simulink model "Rate_Adapating_Testing"  (R2023b)
settings: Solver=FixedStepAuto  StartTime=0.0  StopTime=30  FixedStep=1e-3  RelTol=1e-3  EnableMultiTasking=on
libraries: dspstat3 x3, frdmk64flib x1
settings Model: SimulationMode=external  ExtModeTrigDuration=5  Creator=Jeff  LastModifiedBy=conno
settings SolverCC: AlgebraicLoopSolver=TrustRegion
settings OptimizationCC: EnhancedBackFolding=on  PassReuseOutputArgsAs=Individual arguments  ZeroExternalMemoryAtStartup=off  ZeroInternalMemoryAtStartup=off  MaxStackSize=64  OptimizeBlockOrder=speed  DifferentSizesBufferReuse=on  OptimizationCustomize=off  EfficientTunableParamExpr=on
settings DebuggingCC: ParameterTunabilityLossMsg=error  UnconnectedInputMsg=warning  UnconnectedOutputMsg=warning  UnconnectedLineMsg=warning
settings HardwareCC: ProdBitPerPointer=32  ProdBitPerSizeT=32  ProdBitPerPtrDiffT=32  ProdLargestAtomicInteger=Long  ProdLargestAtomicFloat=Double  ProdWordSize=32  ProdHWDeviceType=ARM Compatible->ARM Cortex
settings ModelReferenceCC: EnableRefExpFcnMdlSchedulingChecks=on
settings SFSimCC: MATLABDynamicMemAlloc=off
settings RTWCC: Description=Embedded Coder  SystemTargetFile=ert.tlc  HardwareBoard=NXP FRDM-K64F  TLCOptions="-aInlineSetEventsForThisBaseRateFcn=TLC_FALSE -aSuppressMultiTaskScheduler=TLC_FALSE  -aRateBasedStepFcn=0"  TemplateMakefile=ert_default_tmf  Toolchain=GNU Tools for ARM Embedded Processors
settings CodeAppCC: ForceParamTrailComments=on  IgnoreCustomStorageClasses=off  OperatorAnnotations=on  SimulinkDataObjDesc=on  SFDataObjDesc=on  InsertBlockDesc=on
settings ERTTargetCC: ExtMode=on  ExtModeTransport=4  ExtModeMexFile=sendToCommService  ExtModeMexArgs='tutorial4_3DM4' 0

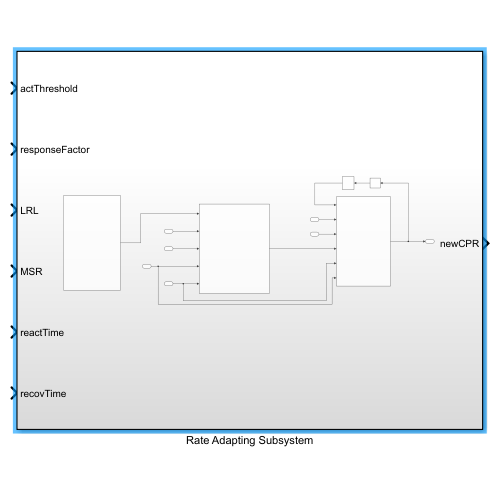
[thumbnail: Simulink's stored preview of the top-level diagram]
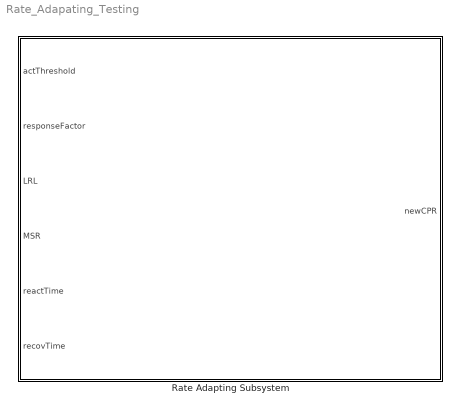
== system Rate_Adapating_Testing ==
  Rate Adapting Subsystem : Subsystem

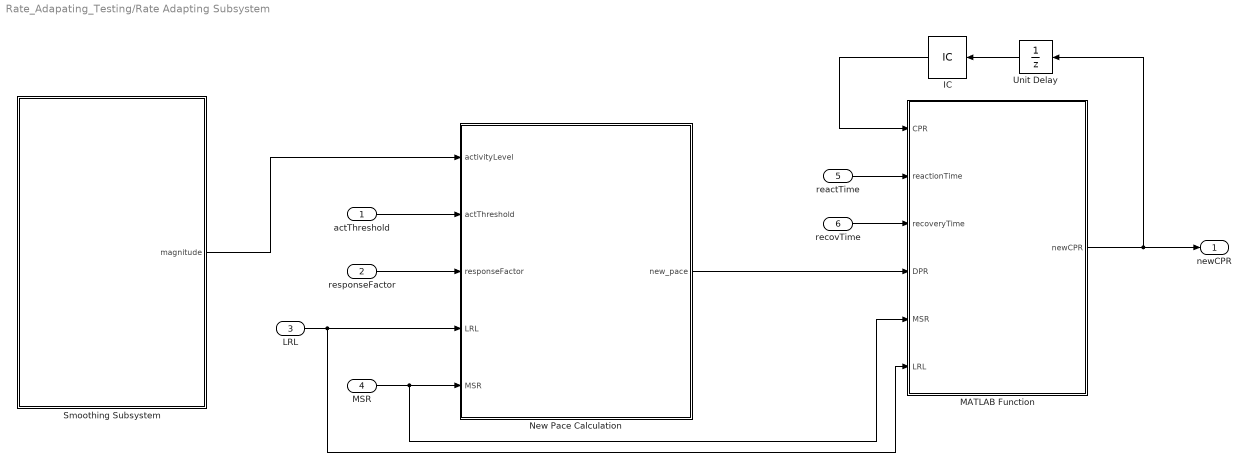
== system Rate_Adapating_Testing/Rate Adapting Subsystem ==
  actThreshold : Inport
  responseFactor : Inport  Port=2
  LRL : Inport  Port=3
  MSR : Inport  Port=4
  reactTime : Inport  Port=5
  recovTime : Inport  Port=6
  IC : InitialCondition  Value=60
  MATLAB Function : MATLAB Function  TreatAsAtomicUnit=on
  New Pace Calculation : MATLAB Function  TreatAsAtomicUnit=on
  Smoothing Subsystem : Subsystem
  Unit Delay : UnitDelay  SampleTime=-1  HasFrameUpgradeWarning=on
  newCPR : Outport
  wires:
  New Pace Calculation/1(new_pace) -> MATLAB Function/4(DPR)
  LRL/1 -> New Pace Calculation/4(LRL), MATLAB Function/6(LRL)
  responseFactor/1 -> New Pace Calculation/3(responseFactor)
  MSR/1 -> New Pace Calculation/5(MSR), MATLAB Function/5(MSR)
  Smoothing Subsystem/1(magnitude) -> New Pace Calculation/1(activityLevel)
  actThreshold/1 -> New Pace Calculation/2(actThreshold)
  MATLAB Function/1(newCPR) -> Unit Delay/1, newCPR/1
  reactTime/1 -> MATLAB Function/2(reactionTime)
  recovTime/1 -> MATLAB Function/3(recoveryTime)
  Unit Delay/1 -> IC/1
  IC/1 -> MATLAB Function/1(CPR)

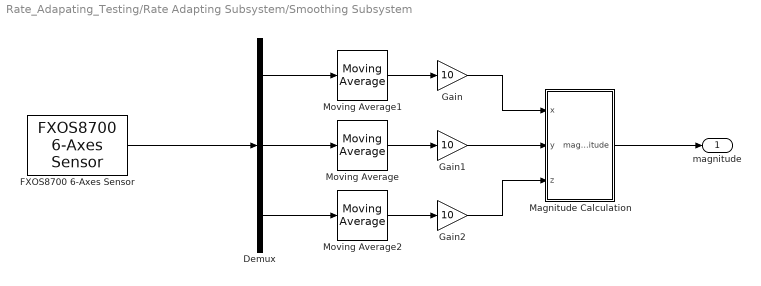
== system Rate_Adapating_Testing/Rate Adapting Subsystem/Smoothing Subsystem ==
  " Magnitude Calculation" : MATLAB Function  TreatAsAtomicUnit=on
  Demux : Demux  Outputs=3
  FXOS8700 6-Axes Sensor : frdmk64flib/FXOS8700 6-Axes Sensor  Activesensor=Accelerometer only  ODR=800Hz  HybridODR=400Hz  Accelfullrange=-4g to +4g  SampleTime=-1
  Gain : Gain  Gain=10
  Gain1 : Gain  Gain=10
  Gain2 : Gain  Gain=10
  Moving Average : dspstat3/Moving Average  Method=Sliding window  ForgettingFactorPort=off  SpecifyWindowLength=on  WindowLength=4  OverlapLength=3  AllowArbitraryInputLength=off  ForgettingFactor=0.9  SimulateUsing=Code generation
  Moving Average1 : dspstat3/Moving Average  Method=Sliding window  ForgettingFactorPort=off  SpecifyWindowLength=on  WindowLength=4  OverlapLength=3  AllowArbitraryInputLength=off  ForgettingFactor=0.9  SimulateUsing=Code generation
  Moving Average2 : dspstat3/Moving Average  Method=Sliding window  ForgettingFactorPort=off  SpecifyWindowLength=on  WindowLength=4  OverlapLength=3  AllowArbitraryInputLength=off  ForgettingFactor=0.9  SimulateUsing=Code generation
  magnitude : Outport
  wires:
  Demux/2 -> Moving Average/1
  Moving Average/1 -> Gain1/1
  Gain/1 -> " Magnitude Calculation"/1(x)
  Demux/1 -> Moving Average1/1
  Gain2/1 -> " Magnitude Calculation"/3(z)
  Moving Average1/1 -> Gain/1
  Demux/3 -> Moving Average2/1
  Gain1/1 -> " Magnitude Calculation"/2(y)
  FXOS8700 6-Axes Sensor/1 -> Demux/1
  Moving Average2/1 -> Gain2/1
  " Magnitude Calculation"/1(magnitude) -> magnitude/1

== matlab function Rate_Adapating_Testing/Rate Adapting Subsystem/New Pace Calculation ==
  data: activityLevel input; actThreshold input; responseFactor input; LRL input; MSR input; new_pace output
function new_pace  = newPace(activityLevel, actThreshold, responseFactor, LRL, MSR)

%Initilization Block
%---------------------------------------------------------------------------------------------------------------------------------------------------
%Acceleration Range of Change
gain = 10; % This is the gain block in the accelorometer
ATMax = sqrt((4*gain)^2+(4*gain)^2+(4*gain)^2)-1; 

%To ensure the pacemaker is static, we remove 1g (gravity)
%Different activity levels listed as strings
actThreshLvl = {'V-Low', 'Low', 'Med-Low', 'Med', 'Med-High', 'High', 'V-High'}; 


%To ensure the percentage is higher than the default 1g, we add 1
%Different activity percentages listed in the same order above
actThreshRange = [0.05*ATMax+1, 0.15*ATMax+1, 0.30*ATMax+1, 0.45*ATMax+1, 0.60*ATMax+1, 0.75*ATMax+1, 0.90*ATMax+1]; 


%This line maps the string levels to the number values in the range
actThreshNum = actThreshRange(find(strcmp(actThreshLvl, char(actThreshold)))); %#ok<FNDSB>
%---------------------------------------------------------------------------------------------------------------------------------------------------



%Condition Block
%---------------------------------------------------------------------------------------------------------------------------------------------------
%condition for if the activity level does not meet the threshold
if(activityLevel <= actThreshNum(1)) 
    new_pace = LRL;


% condition for if the activity level is between the max activity and threshold
elseif(activityLevel > actThreshNum(1) && activityLevel < sqrt(48)) 
    new_pace = (1-exp((-(1/(sqrt(48)-activityLevel)*responseFactor*(activityLevel-actThreshNum(1))))))*(MSR-LRL)+LRL;


%final condition to set the new pace to the max sensor rate if activity level is greater than the max activity
else
    new_pace = MSR; 
%---------------------------------------------------------------------------------------------------------------------------------------------------

end
end

== matlab function Rate_Adapating_Testing/Rate Adapting Subsystem/Smoothing Subsystem/ Magnitude Calculation ==
  data: magnitude output; x input; y input; z input
function magnitude = fcn(x, y, z)
    magnitude = sqrt(x.^2 + y.^2 + z.^2);
end

== matlab function Rate_Adapating_Testing/Rate Adapting Subsystem/MATLAB Function ==
  data: CPR input; reactionTime input; recoveryTime input; DPR input; MSR input; LRL input; newCPR output
function newCPR  = fcn(CPR, reactionTime, recoveryTime, DPR, MSR, LRL)

%Tolerance to prevent value bouncing
tolerance  = 0.05;


if CPR < DPR - tolerance    %Uses Reaction Time

    %Current Time based on Current Pace using inverse function
    currrentTime = -log(1 - (LRL - CPR)/(LRL - MSR))*(reactionTime/11 - 2/11);

    % Increase current time by 1ms
    currrentTime = currrentTime + 0.001;

    %New Current Pace Rate after 1ms increase
    newCPR = (1-exp(-11*currrentTime/(reactionTime-2)))*(MSR-LRL) + LRL;


elseif CPR > DPR + tolerance    %Uses Recovery Time

    %Current Time based on Current Pace using inverse function
    currrentTime = -log((LRL - CPR)/(LRL - MSR))*(recoveryTime/11 - 3/11);
    
    % Increase current time by 1ms
    currrentTime = currrentTime + 0.001;

    %New Current Pace Rate after 1ms increase
    newCPR = (exp(-11*currrentTime/(recoveryTime-3)))*(MSR-LRL) + LRL;

      
else 
    newCPR = CPR; 

end


end
